simulink model "Single_Phase_Full_Control_Bridge_Rectifier_RL_Load"  (R2018a)
settings: Solver=VariableStepAuto  StartTime=0.0  StopTime=0.1  RelTol=1e-3
libraries: powerlib x13, powerlib_meascontrol x4
settings Model: Creator=ozie  LastModifiedBy=ozie

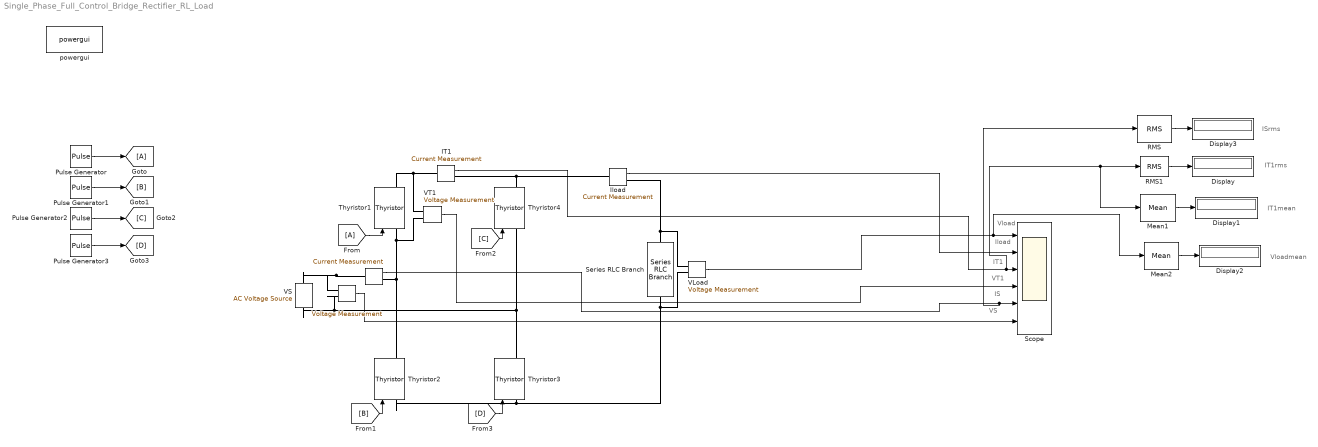
== system Single_Phase_Full_Control_Bridge_Rectifier_RL_Load ==
  note: Vloadmean
  note: IT1mean
  note: IT1rms
  note: ISrms
  note: VS
  note: IS
  note: VT1
  note: IT1
  note: Iload
  note: Vload
  " " : powerlib/Measurements/Voltage Measurement  PhasorSimulation=off  OutputType=Complex  PSBequivalent=0
  " VT1 " : powerlib/Measurements/Voltage Measurement  PhasorSimulation=off  OutputType=Complex  PSBequivalent=0
  "  " : powerlib/Measurements/Current Measurement  PhasorSimulation=off  OutputType=Complex  PSBequivalent=0
  "  Iload " : powerlib/Measurements/Current Measurement  PhasorSimulation=off  OutputType=Complex  PSBequivalent=0
  Display{,1..3} (4 alike) : Display
  IT1 : powerlib/Measurements/Current Measurement  PhasorSimulation=off  OutputType=Complex  PSBequivalent=0
  Mean1 : powerlib_meascontrol/Measurements/Mean  Freq=50  Vinit=0  Ts=0
  Mean2 : powerlib_meascontrol/Measurements/Mean  Freq=50  Vinit=0  Ts=0
  Pulse Generator : DiscretePulseGenerator  PulseType=Time based  Period=1/50  PulseWidth=5  PhaseDelay=(60/360)*1/50
  Pulse Generator1 : DiscretePulseGenerator  PulseType=Time based  Period=0.02  PulseWidth=5  PhaseDelay=(240/360)*1/50
  Pulse Generator2 : DiscretePulseGenerator  PulseType=Time based  Period=0.02  PulseWidth=5  PhaseDelay=(240/360)*1/50
  Pulse Generator3 : DiscretePulseGenerator  PulseType=Time based  Period=0.02  PulseWidth=5  PhaseDelay=(60/360)*1/50
  RMS : powerlib_meascontrol/Measurements/RMS  TrueRMS=on  Freq=50  RMSInit=120  Ts=0
  RMS1 : powerlib_meascontrol/Measurements/RMS  TrueRMS=on  Freq=50  RMSInit=120  Ts=0
  Scope : Scope  NumInputPorts=6
  Series RLC Branch : powerlib/Elements/Series RLC Branch  LConnTagsString=__new0  RConnTagsString=__new0  BranchType=RL  Resistance=8  Inductance=20e-3  SetiL0=off  InitialCurrent=0  Capacitance=1e-6  Setx0=off  InitialVoltage=0  Measurements=None
  Thyristor{1..4} (4 alike) : powerlib/Power Electronics/Thyristor  Ron=0.001  Lon=0  Vf=0.8  IC=0  Rs=500  Cs=250e-9  Measurements=on
  VLoad : powerlib/Measurements/Voltage Measurement  PhasorSimulation=off  OutputType=Complex  PSBequivalent=0
  "VS " : powerlib/Electrical Sources/AC Voltage Source  Amplitude=110*sqrt(2)  Phase=0  Frequency=50  SampleTime=0  Measurements=None  BusType=swing  Pref=10e3  Qref=0  Qmin=-inf  Qmax=+inf
  powergui : powerlib/powergui  Priority=1  SimulationMode=Continuous  SampleTime=50e-6  frequency=60  Iterations=50  frequencyindice=50  Pbase=100e6  ErrMax=1e-4  UnitsV=kV  UnitsW=MW  buscounter=0  FunctionMessages=off  echomessages=off  EnableUseOfTLC=off  CurrentSourceSwitches=off  DisableSnubberDevices=off  DisableRonSwitches=off  DisableVfSwitches=off  DisplayEquations=off  SolverType=Tustin/Backward Euler (TBE)  Interpol=off  ExternalGateDelay=off  methode=off  Ts=100  x0status=blocks  SPID=on  SwTol=0  HookPort=off  RestoreLinks=warning  ResistiveCurrentMeasurement=off  Frange=[0:2:500]  Ylog=off  Xlog=on  ShowGrid=off  save=off  variable=ZData  structure=0  ZoomFFT=off  StartTime=0.0  cycles=1  DisplayStyle=1  fundamental=60  FreqAxis=off  MaxFrequency=1000  frequencyindicesteady=1  RmsSteady=1  display=off
  wires:
  Pulse Generator/1 -> [A]
  [A] -> Thyristor1/1
  Pulse Generator1/1 -> [B]
  [B] -> Thyristor2/1
  [C] -> Thyristor4/1
  Pulse Generator2/1 -> [C]
  Pulse Generator3/1 -> [D]
  [D] -> Thyristor3/1
  VLoad/1 -> Scope/1, Mean2/1
  "  Iload "/1 -> Scope/2
  IT1/1 -> Mean1/1, RMS1/1, Scope/3
  " VT1 "/1 -> Scope/4
  "  "/1 -> RMS/1, Scope/5
  " "/1 -> Scope/6
  Mean2/1 -> Display2/1
  RMS/1 -> Display3/1
  RMS1/1 -> Display/1
  Mean1/1 -> Display1/1
  connections:
  Thyristor1/LConn1 -- " VT1 "/LConn2 -- "  "/RConn1 -- Thyristor2/RConn1
  Thyristor4/LConn1 -- " "/LConn2 -- "VS "/LConn1 -- Thyristor3/RConn1
  Thyristor2/LConn1 -- VLoad/LConn2 -- Series RLC Branch/LConn1 -- Thyristor3/LConn1
  "  Iload "/LConn1 -- IT1/RConn1 -- Thyristor4/RConn1
  "VS "/RConn1 -- "  "/LConn1 -- " "/LConn1
  VLoad/LConn1 -- "  Iload "/RConn1 -- Series RLC Branch/RConn1
  Thyristor1/RConn1 -- " VT1 "/LConn1 -- IT1/LConn1
